simulink model "frequencymeter_simulation_v001"  (R2024b)
settings: Solver=VariableStepAuto  StartTime=0.0  StopTime=10.0  RelTol=1e-3
libraries: ee_lib x3, dspfiltersrcs x2, fl_lib x2
settings Model: Creator=CEYLİN  LastModifiedBy=CEYLİN

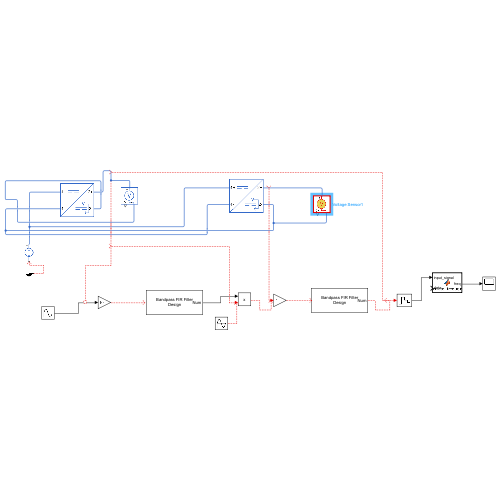
[thumbnail: Simulink's stored preview of the top-level diagram]
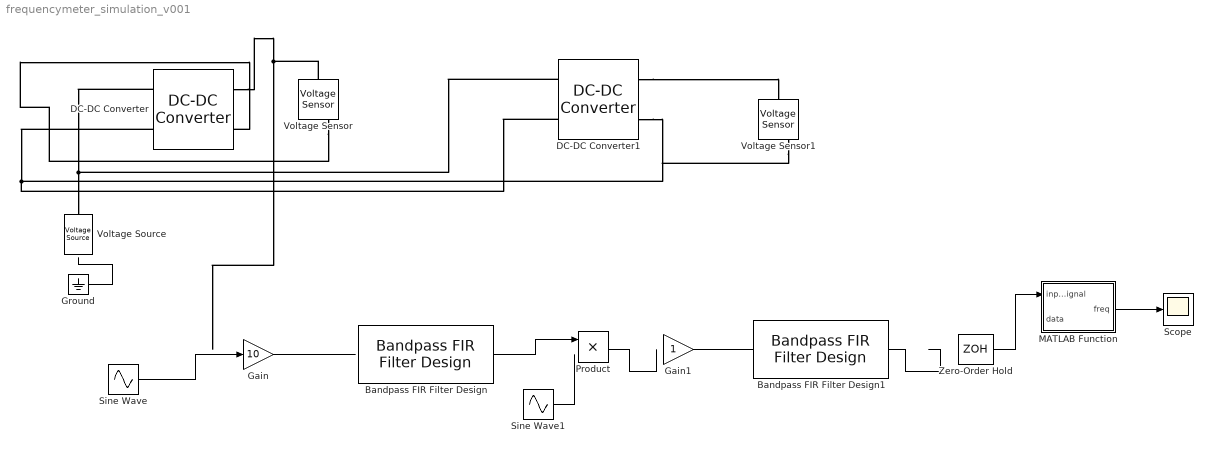
== system frequencymeter_simulation_v001 ==
  Bandpass FIR Filter Design : dspfiltersrcs/Bandpass FIR Filter Design  SmoothParameters=off  SmoothingFactor=0.6  FilterOrderPort=off  FilterOrder=100  MaxOrder=100  CenterFrequencyPort=off  CenterFrequency=0.254  BandwidthPort=off  Bandwidth=0.492  Window=Hamming  SidelobeAttenuationPort=off  SidelobeAttenuation=60  KaiserWindowParameterPort=off  KaiserWindowParameter=.5  OutputDataType=double  SampleTime=-1  SimulateUsing=Interpreted execution
      settings: LibrarySourceBlock=dspfdesign/Bandpass FIR Filter Design
  Bandpass FIR Filter Design1 : dspfiltersrcs/Bandpass FIR Filter Design  SmoothParameters=off  SmoothingFactor=0.6  FilterOrderPort=off  FilterOrder=100  MaxOrder=100  CenterFrequencyPort=off  CenterFrequency=0.0025  BandwidthPort=off  Bandwidth=0.0033  Window=Hamming  SidelobeAttenuationPort=off  SidelobeAttenuation=60  KaiserWindowParameterPort=off  KaiserWindowParameter=.5  OutputDataType=double  SampleTime=-1  SimulateUsing=Interpreted execution
  DC-DC Converter : ee_lib/Semiconductors & Converters/Converters/DC-DC Converter  Vref_option=ee.enum.converters.voltageref.internal  v_ref=5 V  P_rated=10 W  droop_enabled=true  droop_param=ee.enum.converters.droop.value  droop=0.1 V/A  droop_percent=2  Vref_droop=10 V  reversible=ee.enum.converters.directionality.unidirectional  G_diode=1e-8 1/Ohm  P_fixed=1 W  losses_option=ee.enum.converters.lossesOption.proportionalToSquaredCurrent  eff_rated=80  tableOption=ee.enum.converters.lossTableOptionThermal.currentTemp  i_eff_vec=[-2, -1, 1, 2] A  v_eff_vec=[15, 30, 45] V  eff_vec=[66, 76, 80, 74]  eff_2D_table=[66, 66, 66; 76, 76, 76; 80, 80, 80; 74, 74, 74]  model_dynamics=ee.enum.converters.dynamics.no  tau=0.02 s  v_ini=10 V  v1_min=1 V  R1=1000 Ohm  R2=1000 Ohm  fault_condition=ee.enum.faults.faultInputCondition.greaterThan  fault_threshold=0.5  T_eff_vec=[280, 300, 320] K  eff_3D_table=repmat([66; 76; 80; 74], 1, 3, 3)  thermal_mass=100 J/K  initial_temperature=298.15 K
      settings: InternalSimscapePortConfiguration="{\"Bottom\":[],\"Left\":[{\"id\":\"p1\",\"label\":\"1+\",\"type\":\"foundation.electrical.electrical\"},{\"id\":\"n1\",\"label\":\"1-\",\"type\":\"foundation.electrical.electrical\"}],\"Right\":[{\"id\":\"p2\",\"label\":\"2+\",\"type\":\"foundation.electrical.electrical\"},{\"id\":\"n2\",\"label\":\"2-\",\"type\":\"foundation.electrical.electrical\"}],\"Top\":[]}"
  DC-DC Converter1 : ee_lib/Semiconductors & Converters/Converters/DC-DC Converter  Vref_option=ee.enum.converters.voltageref.internal  v_ref=3.3 V  P_rated=10 W  droop_enabled=true  droop_param=ee.enum.converters.droop.value  droop=0.1 V/A  droop_percent=2  Vref_droop=10 V  reversible=ee.enum.converters.directionality.unidirectional  G_diode=1e-8 1/Ohm  P_fixed=1 W  losses_option=ee.enum.converters.lossesOption.proportionalToSquaredCurrent  eff_rated=80  tableOption=ee.enum.converters.lossTableOptionThermal.currentTemp  i_eff_vec=[-2, -1, 1, 2] A  v_eff_vec=[15, 30, 45] V  eff_vec=[66, 76, 80, 74]  eff_2D_table=[66, 66, 66; 76, 76, 76; 80, 80, 80; 74, 74, 74]  model_dynamics=ee.enum.converters.dynamics.no  tau=0.02 s  v_ini=10 V  v1_min=1 V  R1=1000 Ohm  R2=1000 Ohm  fault_condition=ee.enum.faults.faultInputCondition.greaterThan  fault_threshold=0.5  T_eff_vec=[280, 300, 320] K  eff_3D_table=repmat([66; 76; 80; 74], 1, 3, 3)  thermal_mass=100 J/K  initial_temperature=298.15 K
      settings: InternalSimscapePortConfiguration="{\"Bottom\":[],\"Left\":[{\"id\":\"p1\",\"label\":\"1+\",\"type\":\"foundation.electrical.electrical\"},{\"id\":\"n1\",\"label\":\"1-\",\"type\":\"foundation.electrical.electrical\"}],\"Right\":[{\"id\":\"p2\",\"label\":\"2+\",\"type\":\"foundation.electrical.electrical\"},{\"id\":\"n2\",\"label\":\"2-\",\"type\":\"foundation.electrical.electrical\"}],\"Top\":[]}"
  Gain : Gain  Gain=10
  Gain1 : Gain
  Ground : Ground
  MATLAB Function : MATLAB Function  TreatAsAtomicUnit=on
  Product : Product
  Scope : Scope
  Sine Wave : Sin  Frequency=3000000000  SampleTime=0
  Sine Wave1 : Sin  Frequency=3000000000  SampleTime=0
  Voltage Sensor : fl_lib/Electrical/Electrical Sensors/Voltage Sensor
  Voltage Sensor1 : fl_lib/Electrical/Electrical Sensors/Voltage Sensor
  Voltage Source : ee_lib/Sources/Voltage Source  dc_voltage=12 V  ac_voltage=0 V  ac_shift=0 rad  ac_frequency=60 Hz  noise_mode=ee.enum.sources.noise.Disabled  PSD=0 V^2/Hz  sample_time=1e-3 s  repeatability=ee.enum.sources.repeatability.NotRepeatable  user_seed=0  auto_seed=3499211588  i_specify=off  i_priority=None  i=0 A  i_nominal_specify=off  i_nominal_value=1  i_nominal_unit=A  v_specify=off  v_priority=None  v=0 V  v_nominal_specify=off  v_nominal_value=1  v_nominal_unit=V
  Zero-Order Hold : ZeroOrderHold  SampleTime=8.33e-12
  wires:
  Sine Wave/1 -> Gain/1
  Gain/1 -> ?
  Bandpass FIR Filter Design/1 -> Product/1
  ? -> Product/2
  Sine Wave1/1 -> ?
  ? -> Gain1/1
  Product/1 -> ?
  Gain1/1 -> ?
  ? -> Zero-Order Hold/1
  Bandpass FIR Filter Design1/1 -> ?
  Zero-Order Hold/1 -> MATLAB Function/1(input_signal)
  MATLAB Function/1(freq) -> Scope/1
  Ground/1 -> ?
  connections:
  Voltage Sensor/LConn1 -- DC-DC Converter/RConn1
  DC-DC Converter1/RConn1 -- Voltage Sensor1/LConn1
  DC-DC Converter/LConn1 -- Voltage Source/LConn1 -- DC-DC Converter1/LConn1
  DC-DC Converter/LConn2 -- DC-DC Converter1/LConn2 -- DC-DC Converter1/RConn2 -- Voltage Sensor1/RConn2
  Voltage Sensor/RConn2 -- DC-DC Converter/RConn2

== matlab function frequencymeter_simulation_v001/MATLAB Function ==
  data: input_signal input; freq output; data input
function freq = calculate_frequency(input_signal, data)
    fs = 12e9; % Örnekleme frekansı (12 GHz)
    N = length(input_signal); % Sinyal uzunluğu
    fft_result = abs(fft(input_signal)); % FFT sonucu
    [~, idx] = max(fft_result); % Maksimum değer
    freq = (idx - 1) * fs / N; % Frekans hesaplama
end
